simulink model "EE315_Project1_Part3_Model_v2"  (R2013a)
settings: Solver=ode3  StartTime=Time.Start  StopTime=Time.Stop  FixedStep=Time.Step  RelTol=1e-3
values from neighbouring files (symbols this model uses):
  Deq = Dm + 4*Dg*(Nm/Ng)^2+2*De*r^2*(Nm/Ng)^2    (= 1.16977777778)    [EE315_LagCompDesign.m]
  Height = 50    [EE315_LagCompDesign.m]
  J = Jm + 4*Jg*(Nm/Ng)^2+Me*r^2*(Nm/Ng)^2    (= 26.8333333333)    [EE315_LagCompDesign.m]
  kb = (UN-Ra*675)/(825*(2*pi/60))    (= 5.01204959333)    [EE315_LagCompDesign.m]
  kt = 3285/675    (= 4.86666666667)    [EE315_LagCompDesign.m]
  La = 0.92 *10^-3    (= 0.00092)    [EE315_LagCompDesign.m]
  Ng = 1440    [EE315_LagCompDesign.m]
  Nm = 60    [EE315_LagCompDesign.m]
  r = 1    [EE315_LagCompDesign.m]
  Ra = 54.8 *10^-3    (= 0.0548)    [EE315_LagCompDesign.m]
  Tg = (Nm/Ng)*r*Ag*Me    (= 3322.43333333)    [EE315_LagCompDesign.m]
  UN = 470    [EE315_LagCompDesign.m]
undefined symbols (not defined in the file or in its folder): Gc_den, Gc_num, InputRamp_ivel, InputRamp_slope, K, maxCurrentOfMotor, maxMotorDriveInput, maxPosition, SimulinkInputSelector, Time
libraries: simulink x1
settings Model: Creator=Nathansen  LastModifiedBy=Nathansen
settings DataIOCC: SaveOutput=off

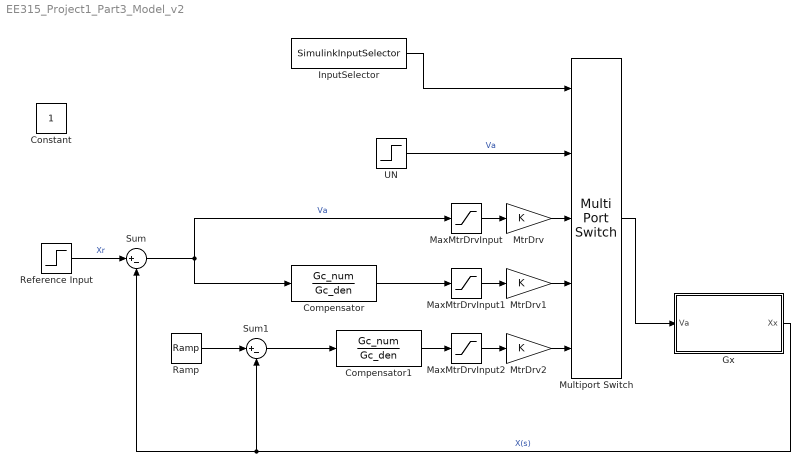
== system EE315_Project1_Part3_Model_v2 ==
  Compensator : TransferFcn  Numerator=Gc_num  Denominator=Gc_den
  Compensator1 : TransferFcn  Numerator=Gc_num  Denominator=Gc_den
  Gx : Subsystem
  InputSelector : Constant  Value=SimulinkInputSelector
  MaxMtrDrvInput : Saturate  UpperLimit=maxMotorDriveInput  LowerLimit=-maxMotorDriveInput
  MaxMtrDrvInput1 : Saturate  UpperLimit=maxMotorDriveInput  LowerLimit=-maxMotorDriveInput
  MaxMtrDrvInput2 : Saturate  UpperLimit=maxMotorDriveInput  LowerLimit=-maxMotorDriveInput
  MtrDrv : Gain  Gain=K
  MtrDrv1 : Gain  Gain=K
  MtrDrv2 : Gain  Gain=K
  Multiport Switch : MultiPortSwitch  Inputs=4
  Ramp : simulink/Sources/Ramp  slope=InputRamp_slope  start=0  X0=InputRamp_ivel
  Reference Input : Step  Time=0  After=Height  SampleTime=Time.Step
  Sum : Sum  Inputs=|+-
  Sum1 : Sum  Inputs=|+-
  UN : Step  Time=0  After=UN  SampleTime=Time.Step
  Constant : Constant  IOType=siggen
  wires:
  Gx/1(Xx) -> Sum/2, Sum1/2  "X(s)"
  Reference Input/1 -> Sum/1  "Xr"
  Sum/1 -> MaxMtrDrvInput/1, Compensator/1  "Va"
  Multiport Switch/1 -> Gx/1(Va)
  UN/1 -> Multiport Switch/2  "Va"
  InputSelector/1 -> Multiport Switch/1
  Sum1/1 -> Compensator1/1
  Ramp/1 -> Sum1/1
  MtrDrv/1 -> Multiport Switch/3
  MtrDrv1/1 -> Multiport Switch/4
  MtrDrv2/1 -> Multiport Switch/5
  Compensator/1 -> MaxMtrDrvInput1/1
  Compensator1/1 -> MaxMtrDrvInput2/1
  MaxMtrDrvInput1/1 -> MtrDrv1/1
  MaxMtrDrvInput/1 -> MtrDrv/1
  MaxMtrDrvInput2/1 -> MtrDrv2/1

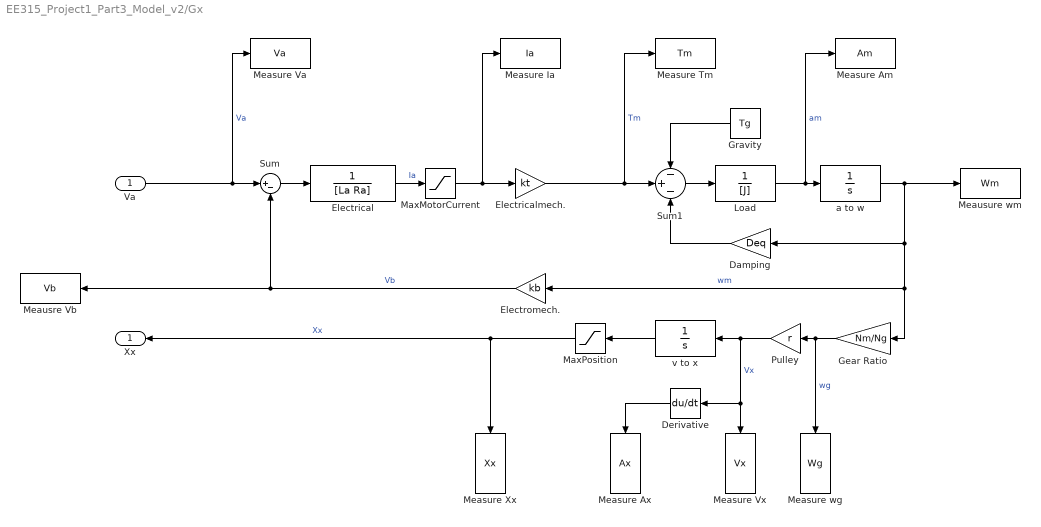
== system EE315_Project1_Part3_Model_v2/Gx ==
  Va : Inport
  Damping : Gain  Gain=Deq
  Derivative : Derivative
  Electrical : TransferFcn  Numerator=1  Denominator=[La Ra]
  "Electricalmech. " : Gain  Gain=kt
  Electromech. : Gain  Gain=kb
  Gear Ratio : Gain  Gain=Nm/Ng
  Gravity : Constant  Value=Tg
  Load : TransferFcn  Numerator=1  Denominator=[J]
  MaxMotorCurrent : Saturate  UpperLimit=maxCurrentOfMotor  LowerLimit=-maxCurrentOfMotor
  MaxPosition : Saturate  UpperLimit=maxPosition  LowerLimit=0
  Measure Ax : ToWorkspace  VariableName=Ax  SampleTime=-1
  Measure Vx : ToWorkspace  VariableName=Vx  SampleTime=-1
  Measure Xx : ToWorkspace  VariableName=Xx  SampleTime=-1
  Measure wg : ToWorkspace  VariableName=Wg  SampleTime=-1
  Measure Am : ToWorkspace  VariableName=Am  SampleTime=-1
  Measure Ia : ToWorkspace  VariableName=Ia  SampleTime=-1
  Measure Tm : ToWorkspace  VariableName=Tm  SampleTime=-1
  Measure Va : ToWorkspace  VariableName=Va  SampleTime=-1
  Meausre Vb : ToWorkspace  VariableName=Vb  SampleTime=-1
  Meausure wm : ToWorkspace  VariableName=Wm  SampleTime=-1
  Pulley : Gain  Gain=r
  Sum : Sum  Inputs=|+-
  Sum1 : Sum  Inputs=-+-
  a to w : TransferFcn  Numerator=1  Denominator=[1 0]
  v to x : TransferFcn  Numerator=1  Denominator=[1 0]
  Xx : Outport
  wires:
  Sum1/1 -> Load/1
  Sum/1 -> Electrical/1
  Electrical/1 -> MaxMotorCurrent/1  "Ia"
  v to x/1 -> MaxPosition/1
  a to w/1 -> Meausure wm/1, Gear Ratio/1, Electromech./1, Damping/1  "wm"
  Gear Ratio/1 -> Measure wg/1, Pulley/1  "wg"
  Damping/1 -> Sum1/3
  Gravity/1 -> Sum1/1
  Pulley/1 -> v to x/1, Derivative/1, Measure Vx/1  "Vx"
  Electromech./1 -> Sum/2, Meausre Vb/1  "Vb"
  Load/1 -> a to w/1, Measure Am/1  "am"
  Va/1 -> Measure Va/1, Sum/1  "Va"
  MaxPosition/1 -> Xx/1, Measure Xx/1  "Xx"
  Derivative/1 -> Measure Ax/1
  "Electricalmech. "/1 -> Measure Tm/1, Sum1/2  "Tm"
  MaxMotorCurrent/1 -> "Electricalmech. "/1, Measure Ia/1
